simulink model "Ejercicio3MotorAcopladoMecanicamente"  (R2016a)
settings: Solver=VariableStepAuto  StartTime=0.0  StopTime=10.0  RelTol=1e-3
values from neighbouring files (symbols this model uses):
  Bm = 0.050    (= 0.05)    [MotorControladoPorArmaduraVariables.m]
  Ea = 270    [MotorControladoPorArmaduraVariables.m]
  Jm = 0.4    [MotorControladoPorArmaduraVariables.m]
  KB = 1    [MotorControladoPorArmaduraVariables.m]
  KT = 1    [MotorControladoPorArmaduraVariables.m]
  La = 0.05    [MotorControladoPorArmaduraVariables.m]
  Ra = 1    [MotorControladoPorArmaduraVariables.m]
  ZL = 4    [MotorControladoPorArmaduraVariables.m]
settings Model: Creator=Abel  LastModifiedBy=Abel

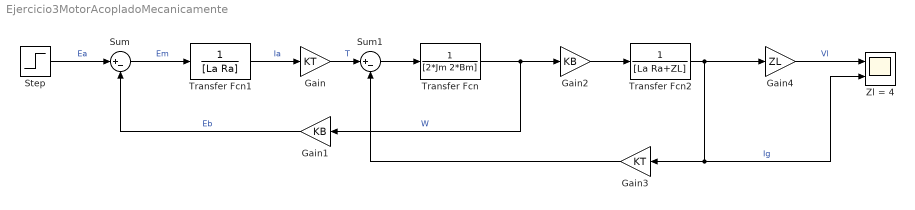
== system Ejercicio3MotorAcopladoMecanicamente ==
  Gain : Gain  Gain=KT
  Gain1 : Gain  Gain=KB
  Gain2 : Gain  Gain=KB
  Gain3 : Gain  Gain=KT
  Gain4 : Gain  Gain=ZL
  Step : Step  After=Ea  SampleTime=0
  Sum : Sum  Inputs=|+-
  Sum1 : Sum  Inputs=|+-
  Transfer Fcn : TransferFcn  Denominator=[2*Jm 2*Bm]
  Transfer Fcn1 : TransferFcn  Denominator=[La Ra]
  Transfer Fcn2 : TransferFcn  Denominator=[La Ra+ZL]
  Zl = 4 : Scope  NumInputPorts=2
  wires:
  Transfer Fcn1/1 -> Gain/1  "Ia"
  Sum/1 -> Transfer Fcn1/1  "Em"
  Gain1/1 -> Sum/2  "Eb"
  Step/1 -> Sum/1  "Ea"
  Transfer Fcn/1 -> Gain1/1, Gain2/1  "W"
  Gain2/1 -> Transfer Fcn2/1
  Gain/1 -> Sum1/1  "T"
  Sum1/1 -> Transfer Fcn/1
  Gain3/1 -> Sum1/2
  Transfer Fcn2/1 -> Gain4/1, Zl = 4/2, Gain3/1  "Ig"
  Gain4/1 -> Zl = 4/1  "Vl"
